simulink subsystem "RT_FlappingDynamic_v1_0"  (R2025a)
settings: Solver=VariableStepAuto  StartTime=0.0  StopTime=30  RelTol=1e-3
undefined symbols (not defined in the file): RT_BEDistFromEffSta_A, RT_BEDistFromHinge_A, RT_BEMassFromHinge_A, RT_BladeFlapInertia_P, RT_HingeFlapPos_P, RT_RotorRadius_P
settings Model: DataDictionary=Rotor.sldd  EnableAccessToBaseWorkspace=off  DefaultTestHarness=FlappingDynamic_v1_0_Harness1  Creator=Admin  LastModifiedBy=Admin

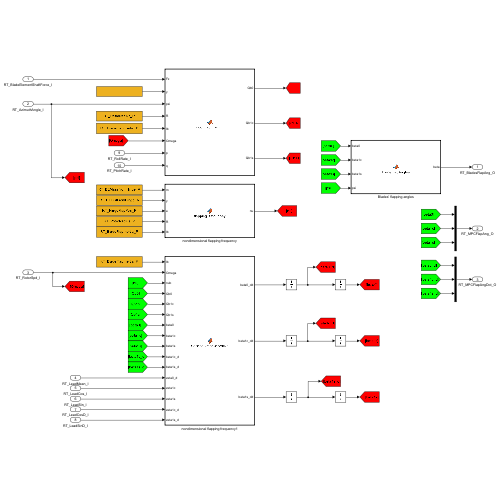
[thumbnail: Simulink's stored preview of the top-level diagram]
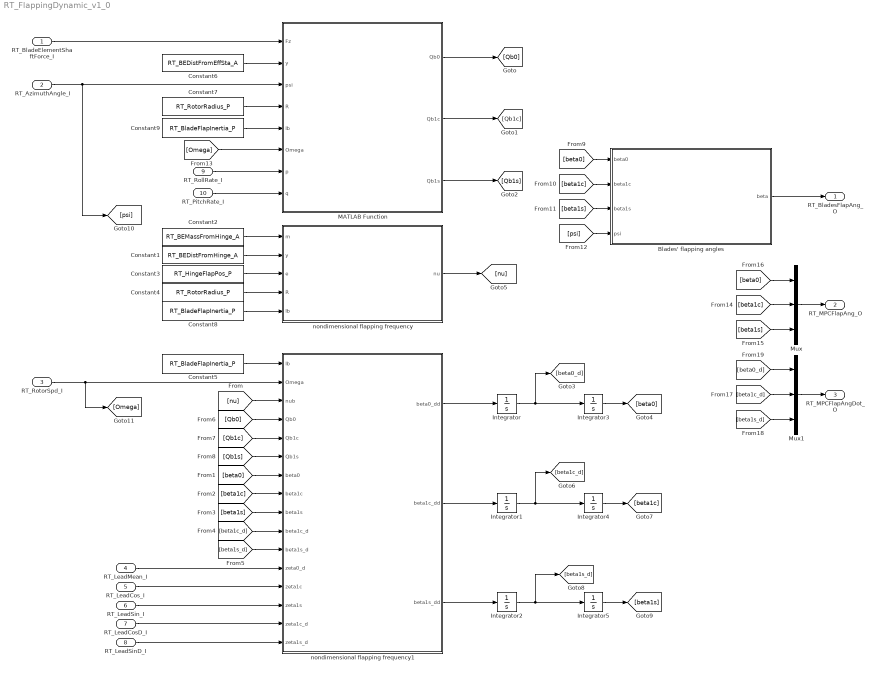
== system RT_FlappingDynamic_v1_0 ==
  RT_BladeElementShaftForce_I : Inport
  RT_AzimuthAngle_I : Inport  Port=2
  RT_RotorSpd_I : Inport  Port=3
  RT_LeadMean_I : Inport  Port=4
  RT_LeadCos_I : Inport  Port=5
  RT_LeadSin_I : Inport  Port=6
  RT_LeadCosD_I : Inport  Port=7
  RT_LeadSinD_I : Inport  Port=8
  RT_RollRate_I : Inport  Port=9
  RT_PitchRate_I : Inport  Port=10
  Blades' flapping angles : MATLAB Function  TreatAsAtomicUnit=on
  Constant1 : Constant  Value=RT_BEDistFromHinge_A
  Constant2 : Constant  Value=RT_BEMassFromHinge_A
  Constant3 : Constant  Value=RT_HingeFlapPos_P
  Constant4 : Constant  Value=RT_RotorRadius_P
  Constant5 : Constant  Value=RT_BladeFlapInertia_P
  Constant6 : Constant  Value=RT_BEDistFromEffSta_A
  Constant7 : Constant  Value=RT_RotorRadius_P
  Constant8 : Constant  Value=RT_BladeFlapInertia_P
  Constant9 : Constant  Value=RT_BladeFlapInertia_P
  Integrator{,1..5} (6 alike) : Integrator
  MATLAB Function : MATLAB Function  TreatAsAtomicUnit=on
  Mux : Mux  Inputs=3
  Mux1 : Mux  Inputs=3
  nondimensional flapping frequency : MATLAB Function  TreatAsAtomicUnit=on
  nondimensional flapping frequency1 : MATLAB Function  TreatAsAtomicUnit=on
  RT_BladesFlapAng_O : Outport
  RT_MPCFlapAng_O : Outport  Port=2
  RT_MPCFlapAngDot_O : Outport  Port=3
  wires:
  MATLAB Function/2(Qb1c) -> [Qb1c]
  MATLAB Function/3(Qb1s) -> [Qb1s]
  nondimensional flapping frequency/1(nu) -> [nu]
  [nu] -> nondimensional flapping frequency1/3(nub)
  nondimensional flapping frequency1/1(beta0_dd) -> Integrator/1
  nondimensional flapping frequency1/2(beta1c_dd) -> Integrator1/1
  nondimensional flapping frequency1/3(beta1s_dd) -> Integrator2/1
  Integrator1/1 -> [beta1c_d], Integrator4/1
  Integrator/1 -> [beta0_d], Integrator3/1
  Integrator2/1 -> [beta1s_d], Integrator5/1
  Integrator3/1 -> [beta0]
  Integrator4/1 -> [beta1c]
  Integrator5/1 -> [beta1s]
  [beta0] -> nondimensional flapping frequency1/7(beta0)
  [beta1c] -> nondimensional flapping frequency1/8(beta1c)
  [beta1s] -> nondimensional flapping frequency1/9(beta1s)
  [beta1c_d] -> nondimensional flapping frequency1/10(beta1c_d)
  [beta1s_d] -> nondimensional flapping frequency1/11(beta1s_d)
  RT_LeadMean_I/1 -> nondimensional flapping frequency1/12(zeta0_d)
  RT_LeadCos_I/1 -> nondimensional flapping frequency1/13(zeta1c)
  RT_LeadSin_I/1 -> nondimensional flapping frequency1/14(zeta1s)
  RT_LeadCosD_I/1 -> nondimensional flapping frequency1/15(zeta1c_d)
  RT_LeadSinD_I/1 -> nondimensional flapping frequency1/16(zeta1s_d)
  Constant5/1 -> nondimensional flapping frequency1/1(Ib)
  RT_RotorSpd_I/1 -> [Omega], nondimensional flapping frequency1/2(Omega)
  Constant6/1 -> MATLAB Function/2(y)
  Constant7/1 -> MATLAB Function/4(R)
  RT_AzimuthAngle_I/1 -> [psi], MATLAB Function/3(psi)
  Constant2/1 -> nondimensional flapping frequency/1(m)
  Constant1/1 -> nondimensional flapping frequency/2(y)
  Constant3/1 -> nondimensional flapping frequency/3(e)
  Constant4/1 -> nondimensional flapping frequency/4(R)
  Constant8/1 -> nondimensional flapping frequency/5(Ib)
  [beta0] -> Blades' flapping angles/1(beta0)
  [beta1c] -> Blades' flapping angles/2(beta1c)
  [beta1s] -> Blades' flapping angles/3(beta1s)
  [psi] -> Blades' flapping angles/4(psi)
  Blades' flapping angles/1(beta) -> RT_BladesFlapAng_O/1
  MATLAB Function/1(Qb0) -> [Qb0]
  RT_BladeElementShaftForce_I/1 -> MATLAB Function/1(Fz)
  [Qb0] -> nondimensional flapping frequency1/4(Qb0)
  [Qb1c] -> nondimensional flapping frequency1/5(Qb1c)
  [Qb1s] -> nondimensional flapping frequency1/6(Qb1s)
  [Omega] -> MATLAB Function/6(Omega)
  Constant9/1 -> MATLAB Function/5(Ib)
  RT_RollRate_I/1 -> MATLAB Function/7(p)
  RT_PitchRate_I/1 -> MATLAB Function/8(q)
  Mux/1 -> RT_MPCFlapAng_O/1
  [beta0] -> Mux/1
  [beta1c] -> Mux/2
  [beta1s] -> Mux/3
  [beta1s_d] -> Mux1/3
  [beta1c_d] -> Mux1/2
  [beta0_d] -> Mux1/1
  Mux1/1 -> RT_MPCFlapAngDot_O/1

== matlab function RT_FlappingDynamic_v1_0/nondimensional flapping frequency ==
  data: m input; nu output; y input; e input; R input; Ib input
function nu  = flapping_frequency(m, y, e, R, Ib)
% m   : [1 x Ns] radial element mass from hinge (kg)
% y   : [1 x Ns]  radial stations from hinge (m)  
% e   : [1 x 1]  hinge ratio with radius (-)
% R   : [1 x 1]  Radius of rotor blade
% Ib  :
% Returns blade flapping natural frequency (N·m)

      
    nu = 1 + e*R/Ib*(m'*y);
end

== matlab function RT_FlappingDynamic_v1_0/nondimensional flapping frequency1 ==
  data: Ib input; Omega input; nub input; Qb0 input; beta0_dd output; Qb1c input; Qb1s input; beta0 input; beta1c input; beta1s input; beta1c_d input; beta1s_d input; zeta0_d input; beta1c_dd output; beta1s_dd output; zeta1c input; zeta1s input; zeta1c_d input; zeta1s_d input
function [beta0_dd, beta1c_dd, beta1s_dd] = SecondOrderDerivative(Ib, Omega, nub, Qb0, Qb1c, Qb1s, beta0, beta1c, beta1s, beta1c_d, beta1s_d, zeta0_d, zeta1c, zeta1s, zeta1c_d, zeta1s_d)
    % Coning acceleration
    beta0_dd = Qb0/Ib - nub * Omega^2 * beta0 + 2 * Omega * beta0 * zeta0_d;
    
    % Longitudinal cyclic flapping acceleration
    beta1c_dd = Qb1c/Ib - 2 * Omega * beta1s_d - (nub-1) * Omega^2 * beta1c + 2 * Omega * beta0 * zeta1c_d - 2 * Omega^2 * beta0 * zeta1s;
    
    % Lateral cyclic flapping acceleration
    beta1s_dd = Qb1s/Ib + 2 * Omega * beta1c_d - (nub-1) * Omega^2 * beta1s + 2 * Omega * beta0 * zeta1s_d + 2 * Omega^2 * beta0 * zeta1c;

end

== matlab function RT_FlappingDynamic_v1_0/Blades' flapping angles ==
  data: beta0 input; beta output; beta1c input; beta1s input; psi input
function beta   = BladeFlapAngles(beta0, beta1c, beta1s, psi)
    
    beta = beta0 + beta1c*cos(psi) + beta1s*sin(psi);
end

== matlab function RT_FlappingDynamic_v1_0/MATLAB Function ==
  data: Fz input; Qb0 output; y input; psi input; Qb1c output; R input; Qb1s output; Ib input; Omega input; p input; q input
function [Qb0, Qb1c, Qb1s] = mbc_flap_forcing(Fz, y, psi, R, Ib, Omega, p, q)
% MBC flap forcing including gyroscopic moment directly in modal form

    Nb = size(Fz, 1);
    psi = psi(:);

    % Aerodynamic blade moment
    Qa = Fz * (y(:) * R);
    % If y is already in meters:
    % Qa = Fz * y(:);

    % Aerodynamic MBC moments
    Qa0  = sum(Qa) / Nb;
    Qa1c = (2 / Nb) * sum(Qa .* cos(psi));
    Qa1s = (2 / Nb) * sum(Qa .* sin(psi));

    % Gyroscopic modal moments
    Qg0  = 0;
    Qg1c = -2 * Ib * Omega * p;
    Qg1s = -2 * Ib * Omega * q;

    % Total MBC moments
    Qb0  = Qa0  + Qg0;
    Qb1c = Qa1c + Qg1c;
    Qb1s = Qa1s + Qg1s;
end
